simulink model "controller_test"  (R2025b)
settings: Solver=VariableStepAuto  StartTime=0.0  StopTime=50  RelTol=1e-3
InitFcn:
  | rng('shuffle')
  | Cl_delta_low = rand - 1;
  | Cl_delta_high = rand + 3;
  | C0_mean = 0.001;
  | C0_bound = 0;
  | C0_low = C0_mean - C0_bound;
  | C0_high = C0_mean + C0_bound;
  | Cl_delta_delay = 0.6 * rand + 0.2;
  | C0_delay = 0.6 * rand + 0.2;
  | step_time = 0.5 * rand + 0.25;
  | step_size = (2*(rand < 0.5)-1) .* (1 + rand);
undefined symbols (not defined in the file or in its folder): gaussian
libraries: simulink x4
settings Model: Creator=finnb  LastModifiedBy=finnb

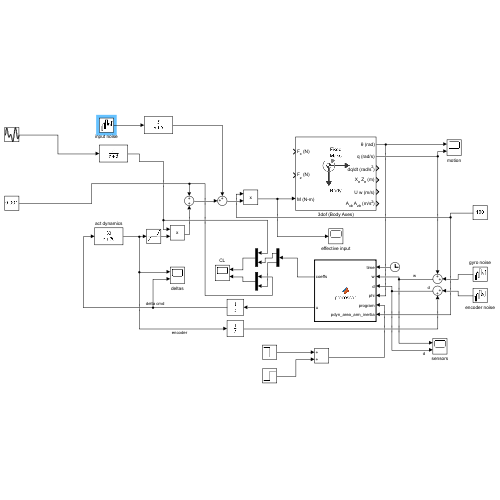
[thumbnail: Simulink's stored preview of the top-level diagram]
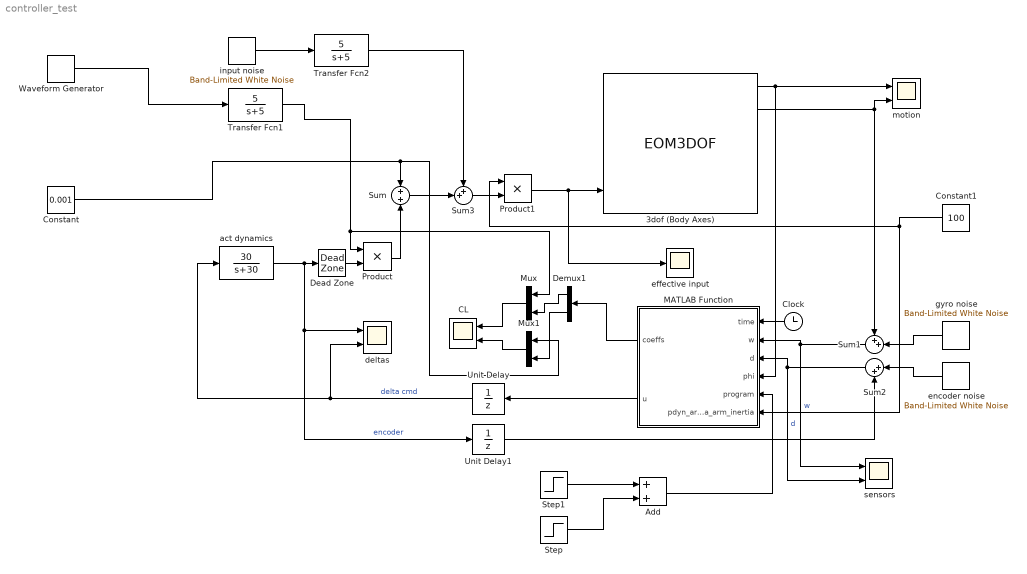
== system controller_test ==
  3dof (Body Axes) : EOM3DOF  v_ini=0  Iyy=1  g=0
  Add : Sum
  CL : Scope  NumInputPorts=2
      settings: ActiveDisplayYMinimum=-0.34401223937761854  ActiveDisplayYMaximum=3.0961101543985672  DataLoggingVariableName=ScopeData2
  Clock : Clock
  Constant : Constant  Value=0.001
  Constant1 : Constant  Value=100
  Dead Zone : DeadZone  LowerValue=-deg2rad(0.5)  UpperValue=deg2rad(0.5)
  Demux1 : Demux  Outputs=2
  MATLAB Function : MATLAB Function  TreatAsAtomicUnit=on
  Mux : Mux  Inputs=2
  Mux1 : Mux  Inputs=2
  Product : Product
  Product1 : Product
  Step : Step  Time=10  SampleTime=0
  Step1 : Step  Time=18  After=-1  SampleTime=0
  Sum : Sum  Inputs=+|+
  Sum1 : Sum  Inputs=++|
  Sum2 : Sum  Inputs=|++
  Sum3 : Sum  Inputs=++|
  Transfer Fcn1 : TransferFcn  Numerator=[5]  Denominator=[1 5]
  Transfer Fcn2 : TransferFcn  Numerator=[5]  Denominator=[1 5]
  Unit Delay : UnitDelay  SampleTime=0.01  HasFrameUpgradeWarning=on
  Unit Delay1 : UnitDelay  SampleTime=0.01  HasFrameUpgradeWarning=on
  Waveform Generator : simulink/Sources/Waveform Generator  OutMin=[]  OutMax=[]  OutDataTypeStr=double  SelectedSignal=1  Signals=2 + sin(0.5, 0.25, 0) + gaussian(0, 0.1, 0010)  BlockNames=MultiportSwitch_bce8c16801a9410  SampleTime=0.1
  act dynamics : TransferFcn  Numerator=[30]  Denominator=[1 30]
  deltas : Scope  NumInputPorts=2
      settings: ActiveDisplayYMinimum=-0.25294237567252237  ActiveDisplayYMaximum=0.25987430109262011  DataLoggingVariableName=ScopeData4
  effective input : Scope
      settings: ActiveDisplayYMinimum=-69.373073038981218  ActiveDisplayYMaximum=58.996374026591177
  encoder noise : simulink/Sources/Band-Limited White Noise  Cov=[1e-8]  Ts=0.01  seed=[23341]
  gyro noise : simulink/Sources/Band-Limited White Noise  Cov=[1e-7]  Ts=0.01  seed=[23341]
  input noise : simulink/Sources/Band-Limited White Noise  Cov=[1e-7]  Ts=0.5  seed=[233]
  motion : Scope  NumInputPorts=2
      settings: ActiveDisplayYMinimum=-0.46681776920388296  ActiveDisplayYMaximum=1.811334987780544
  sensors : Scope  NumInputPorts=2
      settings: ActiveDisplayYMinimum=-1.8974174144580771  ActiveDisplayYMaximum=2.1283724957411052  DataLoggingVariableName=ScopeData3
  wires:
  Unit Delay/1 -> act dynamics/1, deltas/2  "delta cmd"
  Sum3/1 -> Product1/2
  3dof (Body Axes)/2 -> Sum1/1, motion/2
  Clock/1 -> MATLAB Function/1(time)
  Sum1/1 -> sensors/1, MATLAB Function/2(w)  "w"
  Sum2/1 -> MATLAB Function/3(d), sensors/2  "d"
  Sum/1 -> Sum3/2
  input noise/1 -> Transfer Fcn2/1
  Product1/1 -> effective input/1, 3dof (Body Axes)/3
  3dof (Body Axes)/1 -> MATLAB Function/4(phi), motion/1
  Unit Delay1/1 -> Sum2/2
  Step/1 -> Add/2
  Step1/1 -> Add/1
  Add/1 -> MATLAB Function/5(program)
  act dynamics/1 -> Dead Zone/1, Unit Delay1/1, deltas/1  "encoder"
  Dead Zone/1 -> Product/2
  Transfer Fcn2/1 -> Sum3/1
  Constant/1 -> Mux1/1, Sum/1
  Product/1 -> Sum/2
  Transfer Fcn1/1 -> Mux/1, Product/1
  MATLAB Function/1(coeffs) -> Demux1/1
  Demux1/2 -> Mux1/2
  Demux1/1 -> Mux/2
  Mux1/1 -> CL/2
  Mux/1 -> CL/1
  encoder noise/1 -> Sum2/1
  gyro noise/1 -> Sum1/2
  MATLAB Function/2(u) -> Unit Delay/1
  Waveform Generator/1 -> Transfer Fcn1/1
  Constant1/1 -> MATLAB Function/6(pdyn_area_arm_inertia), Product1/1

== matlab function controller_test/MATLAB Function ==
  settings: updateMethod=DISCRETE  sampleTime=0.01
  data: time input; w input; coeffs output; d input; phi input; u output; program input; pdyn_area_arm_inertia input
function [coeffs, u] = processor(time, w, d, phi, program, pdyn_area_arm_inertia)
    % p : parameters
    % r : regressors
    % w : angular rate measurement
    % d : canard angle measurement / command
    % pdyn_area_arm_inertia : everything in L except coefficients. match with gain in sim

    L_min = 0.1; % limit roll control derivative for low authority conditions
    u_max = deg2rad(15); 

    if abs(d) <= deg2rad(1)
        d = 0;
    end
    
    [C_l_delta, C_l_0] = controller_estimator(time, w, d, pdyn_area_arm_inertia);
    coeffs = [C_l_delta, C_l_0];

    L_delta = C_l_delta * pdyn_area_arm_inertia;
    L_delta = 1 / (max(min(1/L_delta, 1/L_min), -1/L_min)); % lower bounds

    u = controller_law([phi; w], program, L_delta);
    u = min(max(u, -u_max), u_max); % upper bounds

end
